simulink model "ipmsm_current_control_CV_FF"  (R2023a)
settings: Solver=FixedStepDiscrete  StartTime=0.0  StopTime=0.8  FixedStep=Ts  RelTol=1e-3  EnableMultiTasking=on
PreLoadFcn:
  | ee_ipmsm_velocity_control_data;
StopFcn:
  | ee_addSimlogTimeStamp(bdroot)
values from neighbouring files (symbols this model uses):
  ActCV = 1    [ipmsm_current_control_data.m]
  down1 = den(1)    [ipmsm_current_control_data.m]
  down2 = den(2)    [ipmsm_current_control_data.m]
  Ki_id = 0.6*Ld/(5*sigma*sigma)    (= 3750)    [ipmsm_current_control_data.m]
  Ki_iq = 0.6*Lq/(5*sigma*sigma)    (= 3750)    [ipmsm_current_control_data.m]
  Kp_id = 0.6*Ld/sigma    (= 1.5)    [ipmsm_current_control_data.m]
  Kp_iq = 0.6*Lq/sigma    (= 1.5)    [ipmsm_current_control_data.m]
  Ld = 0.2e-3    (= 0.0002)    [ipmsm_current_control_data.m]
  Lq = 0.2e-3    (= 0.0002)    [ipmsm_current_control_data.m]
  p = 4    [ipmsm_current_control_data.m]
  Pmax = 1.2*445.3845    (= 534.4614)    [ipmsm_current_control_data.m]
  psim = 0.0064    [ipmsm_current_control_data.m]
  Tmax = 1.2*0.8223    (= 0.98676)    [ipmsm_current_control_data.m]
  Ts = 1e-6    (= 1e-06)    [ipmsm_current_control_data.m]
  Tsi = 5e-5    (= 5e-05)    [ipmsm_current_control_data.m]
  up = num(2)    [ipmsm_current_control_data.m]
  Vnom = 24    [ipmsm_current_control_data.m]
undefined symbols (not defined in the file or in its folder): ee_sli_rtmsupport, gcbh, ID_MAP, IQ_MAP, RPM_VECT, TQ_VECT, VDC_VECT
libraries: nesl_utility x13, fl_lib x10, simulink x10, ee_lib x5, spsMeanLib x4, slpidlib x2, eeDiscretePi x2, eeTransforms x2, eeVelocityController x1, eePwmGeneratorTwoLevel x1, SignalEditorBlockLib x1
(part 1 of 2)
CloseFcn:
  | try,close(h1_ee_ipmsm_velocity_control),end
  | clear h1_ee_ipmsm_velocity_control
  | 
  | clear simlog_ee_ipmsm_velocity_control
  | clear logsout_ee_ipmsm_velocity_control
  | 
  | clear Pmax Tmax p psim Ld Lq L0 Rs Jm
  | clear Cdc Vnom V1 AH0
  | clear Ts fsw Tsi Tso Kp_id Ki_id Kp_iq Ki_iq
  | clear numd_id dend_id numd_iq dend_iq
  | clear Kp_omega Ki_omega numd_omega dend_omega
  | clear ID_MAP IQ_MAP RPM_VECT TQ_VECT VDC_VECT
Description:
  | IPMSM Velocity Control
settings Model: SimulationMode=accelerator  Creator=The MathWorks, Inc.  LastModifiedBy=zxzhu
settings SolverCC: AlgebraicLoopSolver=TrustRegion  AutoInsertRateTranBlk=on  MaxZcPerStep=1
settings DataIOCC: MaxDataPoints=210000  ReturnWorkspaceOutputs=off  SignalLoggingName=logsout_ee_ipmsm_velocity_control
settings OptimizationCC: ReuseModelBlockBuffer=off  LifeSpan=inf
settings DebuggingCC: UnderspecifiedInitializationDetection=Classic  MergeDetectMultiDrivingBlocksExec=none  UnconnectedInputMsg=warning  UnconnectedOutputMsg=warning  UnconnectedLineMsg=warning  SFUnexpectedBacktrackingDiag=warning  SFNoUnconditionalDefaultTransitionDiag=warning  SFExecutionAtInitializationDiag=none  ArithmeticOperatorsInVariantConditions=warning
settings ModelReferenceCC: EnableRefExpFcnMdlSchedulingChecks=on
settings SFSimCC: SimUseLocalCustomCode=off  CustomCodeUndefinedFunction=UseInterfaceOnly
settings RTWCC: RTWUseLocalCustomCode=off  DLArmComputeVersion=19.05
settings CodeAppCC: StateflowObjectComments=on
settings GRTTargetCC: TargetLangStandard=C89/C90 (ANSI)
settings ConfigComp: CovMetricSettings=dw  CovSaveCumulativeToWorkspaceVar=on  CovSaveSingleToWorkspaceVar=on  CovExternalEMLEnable=off
settings SimscapeCC: SimscapeNormalizeSystem=off  SimscapeLogType=all  SimscapeLogSimulationStatistics=on  SimscapeLogName=simlog_ee_ipmsm_velocity_control  SimscapeLogDataHistory=210000

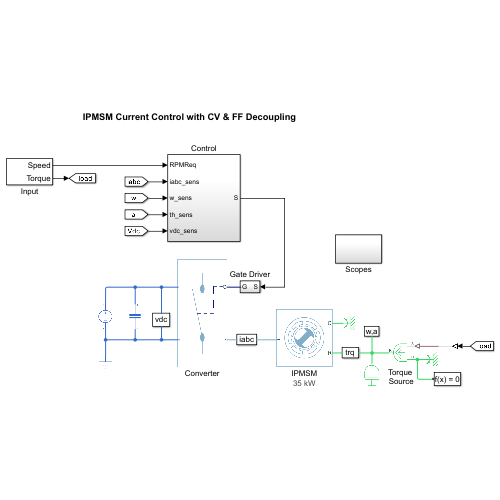
[thumbnail: Simulink's stored preview of the top-level diagram]
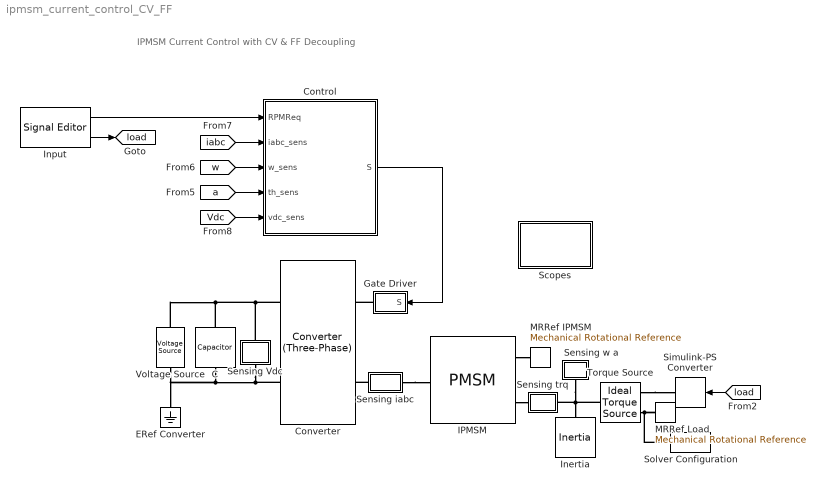
== system ipmsm_current_control_CV_FF ==
  note: IPMSM Current Control with CV & FF Decoupling
  C : fl_lib/Electrical/Electrical Elements/Capacitor  c=Cdc F  r=1e-6 Ohm  g=0 1/Ohm  i_specify=off  i_priority=None  i=0 A  i_nominal_specify=off  i_nominal_unit=A  i_nominal_value=1  v_specify=off  v_priority=None  v=0 V  v_nominal_specify=off  v_nominal_unit=V  v_nominal_value=1  vc_specify=on  vc_priority=None  vc=Vnom V  vc_nominal_specify=off  vc_nominal_unit=V  vc_nominal_value=1
  Control : Subsystem
  Converter : ee_lib/Semiconductors & Converters/Converters/Converter (Three-Phase)  port_option=ee.enum.threePhasePort.composite  device_type=3  K=0  Vf=0.8 V  Ron=0.001 Ohm  Rds=0.001 Ohm  Goff=1e-5 1/Ohm  Vgt=1 V  Vgt_off=-1 V  Ih=1 A  Vth=0.5 V  diode_param=2  diode_Vf=0.8 V  diode_Ron=0.001 Ohm  diode_Goff=1e-5 1/Ohm  diode_C=50 nF  diode_iRM=-235 A  diode_iF=300 A  diode_idot=-50 A/us  diode_trr_param=1  diode_trr_factor=3  diode_trr=15 us  diode_Qrr=1.5e+3 s*uA  snubber_type=0  Cs=1e-7 F  Rs=0.1 Ohm
  ERef Converter : fl_lib/Electrical/Electrical Elements/Electrical Reference
  Gate Driver : Subsystem
  IPMSM : ee_lib/Electromechanical/Permanent Magnet/PMSM  port_option=ee.enum.threePhasePort.composite  winding_type=ee.enum.statorconnection.wye  machine_param=ee.enum.pmsm.parameterization.constant  nPolePairs=p  pmflux_param=1  pm_flux_linkage=psim Wb  torque_constant=0.18 N*m/A  back_emf_constant=0.18 V/(rad/s)  stator_param=1  Ld=Ld H  Lq=Lq H  idVec=[-200, 0, 200] A  iqVec=[-200, 0, 200] A  LdMatrix=0.0002 * ones(3, 3) H  LqMatrix=0.0002 * ones(3, 3) H  PmMatrix=0.1 * ones(3, 3) Wb  ktMatrix=0.18 * ones(3, 3) N*m/A  keMatrix=0.18 * ones(3, 3) V/(rad/s)  L0=L0 H  Ls=0.0002 H  Lm=0.00002 H  Ms=0.00002 H  Rs=Rs Ohm  zero_sequence=ee.enum.park.zerosequence.exclude  axes_param=ee.enum.rotorangle.daxis  loss_param=ee.enum.ironloss.none  losses_oc=[0, 0, 0] W  losses_sc=[0, 0, 0] W  f_losses=60 Hz  Isc_losses=95 A  J=0 kg*m^2  lam=0 N*m/(rad/s)  i_d_specify=off  i_d_priority=None  i_d=0 A  i_d_nominal_specify=off  i_d_nominal_unit=A  i_d_nominal_value=1  i_q_specify=off  i_q_priority=None  i_q=0 A  i_q_nominal_specify=off  i_q_nominal_unit=A  i_q_nominal_value=1  torque_specify=off  torque_priority=None  torque=0 N*m  torque_nominal_specify=off  torque_nominal_unit=N*m  torque_nominal_value=1  angular_velocity_specify=on  angular_velocity_priority=None  angular_velocity=0 rpm  angular_velocity_nominal_specify=off  angular_velocity_nominal_unit=rpm  angular_velocity_nominal_value=1  angular_position_specify=on  angular_position_priority=High  angular_position=0 rad  angular_position_nominal_specify=off  angular_position_nominal_unit=deg  angular_position_nominal_value=1  alpha=3.93e-3 1/K  alpha_flux=-0.001 1/K  Tmeas=298.15 K  stator_thermal_mass=100 J/K  rotor_thermal_mass=200 J/K  Rm_percent_rotor=90  Rd_percent_rotor=30  temperatureA_specify=off  temperatureA_priority=High  temperatureA=25 degC  temperatureA_nominal_specify=off  temperatureA_nominal_unit=degC  temperatureA_nominal_value=1  temperatureB_specify=off  temperatureB_priority=High  temperatureB=25 degC  temperatureB_nominal_specify=off  temperatureB_nominal_unit=degC  temperatureB_nominal_value=1  temperatureC_specify=off  temperatureC_priority=High  temperatureC=25 degC  temperatureC_nominal_specify=off  temperatureC_nominal_unit=degC  temperatureC_nominal_value=1  temperatureR_specify=off  temperatureR_priority=High  temperatureR=25 degC  temperatureR_nominal_specify=off  temperatureR_nominal_unit=degC  temperatureR_nominal_value=1
      settings: AttributesFormatString=35 kW  InternalSimscapePortConfiguration="{\"Bottom\":[],\"Left\":[{\"id\":\"N\",\"label\":\"~\",\"type\":\"foundation.electrical.three_phase\"}],\"Right\":[{\"id\":\"R\",\"label\":\"R\",\"type\":\"foundation.mechanical.rotational.rotational\"},{\"id\":\"C\",\"label\":\"C\",\"type\":\"foundation.mechanical.rotational.rotational\"}],\"Top\":[]}"
  Inertia : fl_lib/Mechanical/Rotational Elements/Inertia  inertia=Jm kg*m^2  num_ports=foundation.enum.numPorts2.one  w_specify=on  w_priority=High  w=0 rpm  w_nominal_specify=off  w_nominal_unit=rad/s  w_nominal_value=1  t_specify=off  t_priority=High  t=0 N*m  t_nominal_specify=off  t_nominal_unit=N*m  t_nominal_value=1
  Input : SignalEditorBlockLib/Signal Editor  FileName=ipmsm_current_control_Input.mat  ActiveScenario=Test_2000rpm  ActiveSignal=Speed  IsBus=off  OutputBusObjectStr=Bus: BusObject  SampleTime=0  OutputAfterFinalValue=Extrapolation  Unit=inherit  PreserveSignalName=on  ApplySigPropsToAllScenarios=on
  MRRef IPMSM : fl_lib/Mechanical/Rotational Elements/Mechanical Rotational Reference
  MRRef Load : fl_lib/Mechanical/Rotational Elements/Mechanical Rotational Reference
  Scopes : Subsystem
  Sensing Vdc : Subsystem
      mask Display: disp('vdc')
  Sensing trq : Subsystem
      mask Display: disp('trq')
  Sensing w a : Subsystem
      mask Display: disp('w,a')
  Sensing iabc : Subsystem
      mask Display: disp('iabc')
  Simulink-PS Converter : nesl_utility/Simulink-PS Converter  PhysicalDomain=network_engine_domain  SubClassName=ps_input  LeftPortType=input  RightPortType=output  PseudoPeriodic=off  Frequencies=[]  NoiseDistribution=none  NoiseParameters=[]  Unit=N*m  AffineConversion=off  FilteringAndDerivatives=zero  SimscapeFilterOrder=1  InputFilterTimeConstant=0.001  UdotUserProvided=1
  Solver Configuration : nesl_utility/Solver Configuration  PhysicalDomain=network_engine_domain  SubClassName=solver  LeftPortType=input  RightPortType=generic  Tones=[]  Harmonics=[]  SimulateNoise=off  Profile=off  UseLocalSampling=off  EnableSwitchedLinearOptims=on  FrequencyDomain=off  UseCCode=off  RelTol=0.001  AbsTol=1e-06  MinStep=1e-09  ToWorkspace=off  RevertToSquareIcSolve=off  NumHomotopyIterations=100  PhasorMode=off  PhasorModeNumHarmonics=1  ConsistencySolver=NEWTON_FTOL  IndexReductionMethod=DerivativeReplacement  DoDC=off  ResidualTolerance=1e-9  ConsistencyTolSource=GLOBAL  ConsistencyAbsTol=0.001  ConsistencyRelTol=0.001  ConsistencyTolFactor=0.001  UseLocalSolver=on  LocalSolverChoice=NE_BACKWARD_EULER_ADVANCER  ResolveIndetEquations=on  FunctionEvalNumThread=1  LocalSolverSampleTime=Ts  DoFixedCost=on  MaxNonlinIter=5  MaxModeIter=2  ComputeImpulses=off  ImpulseIterations=2  LinearAlgebra=auto  LinearAlgebraNumThread=0  EquationFormulation=NE_TIME_EF  DelaysMemoryBudget=1024  AutomaticFiltering=on  FilteringTimeConstant=0.001  PartitionStorageMethod=AS_NEEDED  PartitionMemoryBudget=1024  PartitionMethod=FAST
  Torque Source : fl_lib/Mechanical/Mechanical Sources/Ideal Torque Source
  Voltage Source : ee_lib/Sources/Voltage Source  dc_voltage=Vnom V  ac_voltage=0 V  ac_shift=0 rad  ac_frequency=60 Hz  noise_mode=ee.enum.sources.noise.Disabled  PSD=0 V^2/Hz  sample_time=1e-3 s  repeatability=ee.enum.sources.repeatability.NotRepeatable  user_seed=0  auto_seed=3499211588  i_specify=off  i_priority=None  i=0 A  i_nominal_specify=off  i_nominal_unit=A  i_nominal_value=1  v_specify=off  v_priority=None  v=0 V  v_nominal_specify=off  v_nominal_unit=V  v_nominal_value=1
  tag scope: load=global
  wires:
  Control/1(S) -> Gate Driver/1(S)
  [load] -> Simulink-PS Converter/1
  [Vdc] -> Control/5(vdc_sens)
  [iabc] -> Control/2(iabc_sens)
  [w] -> Control/3(w_sens)
  [a] -> Control/4(th_sens)
  Input/2 -> [load]
  Input/1 -> Control/1(RPMReq)
  connections:
  Converter/RConn1 -- Sensing Vdc/LConn1 -- Voltage Source/LConn1 -- C/LConn1
  Torque Source/LConn1 -- Sensing trq/RConn1 -- Inertia/LConn1 -- Sensing w a/LConn1
  Gate Driver/RConn1 -- Converter/LConn1
  Torque Source/RConn1 -- Simulink-PS Converter/RConn1
  Torque Source/RConn2 -- Solver Configuration/RConn1 -- MRRef Load/LConn1
  Sensing iabc/LConn1 -- Converter/LConn2
  IPMSM/RConn2 -- MRRef IPMSM/LConn1
  IPMSM/RConn1 -- Sensing trq/LConn1
  Voltage Source/RConn1 -- ERef Converter/LConn1 -- Converter/RConn2 -- Sensing Vdc/RConn1 -- C/RConn1
  Sensing iabc/RConn1 -- IPMSM/LConn1

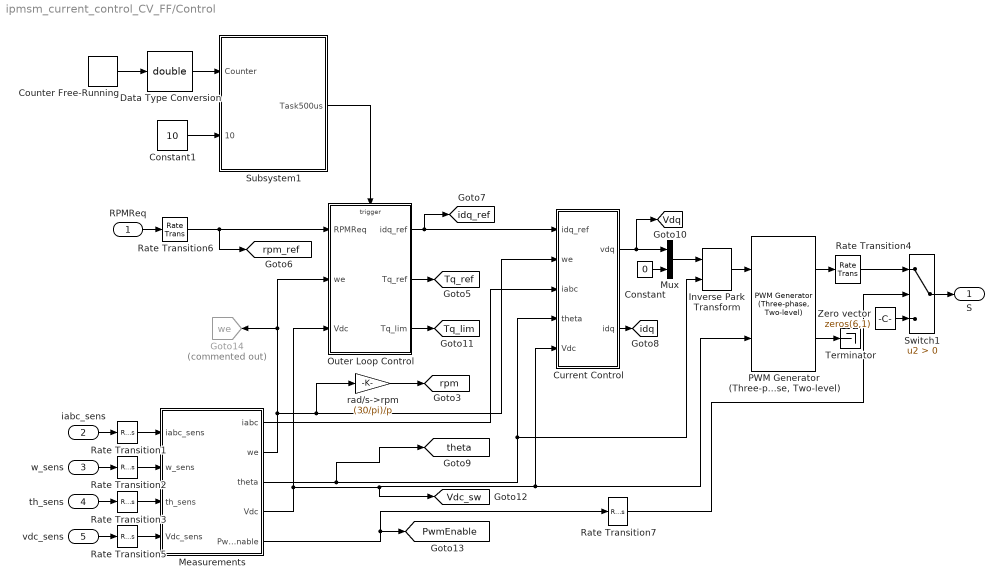
== system ipmsm_current_control_CV_FF/Control ==
  RPMReq : Inport
  iabc_sens : Inport  Port=2
  w_sens : Inport  Port=3
  th_sens : Inport  Port=4
  vdc_sens : Inport  Port=5
  Constant : Constant  Value=0  SampleTime=-1
  Constant1 : Constant  Value=10
  Counter Free-Running : simulink/Sources/Counter Free-Running  NumBits=32  tsamp=5e-5
  Current Control : Subsystem
  Data Type Conversion : DataTypeConversion  OutDataTypeStr=double  SaturateOnIntegerOverflow=off  RndMeth=Floor
  Goto14 : Goto  Commented=on  GotoTag=we  TagVisibility=global
  Inverse Park Transform : eeTransforms/Inverse Park Transform  AxisAlignment=D-axis  PowerInvariant=off
  Measurements : Subsystem
  Mux : Mux  Inputs=2
  Outer Loop Control : Subsystem
  "PWM Generator (Three-phase, Two-level)" : eePwmGeneratorTwoLevel/PWM Generator (Three-phase, Two-level)  PWMMode=Continuous PWM (CPWM)  CPWMMode=SVM: space vector modulation  DPWMMode=60 DPWM: 60 degree discontinuous PWM  fsw=fsw  Ts=Ts
      settings: SamplingMode=Asymmetric
  Rate Transition{1..7} (7 alike) : RateTransition
  Subsystem1 : Subsystem
  Switch1 : Switch  Criteria=u2 > Threshold  SaturateOnIntegerOverflow=off  InputSameDT=off
  Terminator : Terminator
  Zero vector : Constant  Value=zeros(6,1)
  rad/s->rpm : Gain  Gain=(30/pi)/p
  S : Outport  VectorParamsAs1DForOutWhenUnconnected=off
  tag scope: PwmEnable=global, Tq_lim=global, Tq_ref=global, Vdc_sw=global, Vdq=global, idq=global, idq_ref=global, rpm=global, rpm_ref=global, theta=global
  wires:
  Current Control/1(vdq) -> Mux/1, [Vdq]
  Measurements/1(iabc) -> Current Control/3(iabc)
  "PWM Generator (Three-phase, Two-level)"/1 -> Rate Transition4/1
  iabc_sens/1 -> Rate Transition1/1
  w_sens/1 -> Rate Transition2/1
  th_sens/1 -> Rate Transition3/1
  vdc_sens/1 -> Rate Transition5/1
  Outer Loop Control/1(idq_ref) -> [idq_ref], Current Control/1(idq_ref)
  RPMReq/1 -> Rate Transition6/1
  "PWM Generator (Three-phase, Two-level)"/2 -> Terminator/1
  Rate Transition1/1 -> Measurements/1(iabc_sens)
  Rate Transition2/1 -> Measurements/2(w_sens)
  Rate Transition3/1 -> Measurements/3(th_sens)
  Rate Transition5/1 -> Measurements/4(Vdc_sens)
  Rate Transition6/1 -> [rpm_ref], Outer Loop Control/1(RPMReq)
  Measurements/4(Vdc) -> Outer Loop Control/3(Vdc), [Vdc_sw], Current Control/5(Vdc), "PWM Generator (Three-phase, Two-level)"/2
  Outer Loop Control/2(Tq_ref) -> [Tq_ref]
  Measurements/2(we) -> Goto14/1, Outer Loop Control/2(we), Current Control/2(we), rad/s->rpm/1
  rad/s->rpm/1 -> [rpm]
  Current Control/2(idq) -> [idq]
  Outer Loop Control/3(Tq_lim) -> [Tq_lim]
  Switch1/1 -> S/1
  Rate Transition4/1 -> Switch1/1
  Measurements/5(PwmEnable) -> Rate Transition7/1, [PwmEnable]
  Zero vector/1 -> Switch1/3
  Rate Transition7/1 -> Switch1/2
  Mux/1 -> Inverse Park Transform/1
  Constant/1 -> Mux/2
  Constant1/1 -> Subsystem1/2(10)
  Counter Free-Running/1 -> Data Type Conversion/1
  Subsystem1/1(Task500us) -> Outer Loop Control/Trigger
  Data Type Conversion/1 -> Subsystem1/1(Counter)
  Inverse Park Transform/1 -> "PWM Generator (Three-phase, Two-level)"/1
  Measurements/3(theta) -> Current Control/4(theta), Inverse Park Transform/2, [theta]

== system ipmsm_current_control_CV_FF/Gate Driver ==
  S : Inport
  Demux : Demux  Outputs=6
  Simulink-PS Converter{1..6} (6 alike) : nesl_utility/Simulink-PS Converter  PhysicalDomain=network_engine_domain  SubClassName=ps_input  LeftPortType=input  RightPortType=output  PseudoPeriodic=off  Frequencies=[]  NoiseDistribution=none  NoiseParameters=[]  Unit=1  AffineConversion=off  FilteringAndDerivatives=zero  SimscapeFilterOrder=1  InputFilterTimeConstant=0.001  UdotUserProvided=1
  Six-Pulse Gate Multiplexer : ee_lib/Semiconductors & Converters/Converters/Six-Pulse Gate Multiplexer  port_option=ee.enum.controlport.ps
  G : PMIOPort  Side=Right
  wires:
  Demux/1 -> Simulink-PS Converter1/1
  S/1 -> Demux/1
  Demux/4 -> Simulink-PS Converter4/1
  Demux/2 -> Simulink-PS Converter2/1
  Demux/3 -> Simulink-PS Converter3/1
  Demux/5 -> Simulink-PS Converter5/1
  Demux/6 -> Simulink-PS Converter6/1
  connections:
  Six-Pulse Gate Multiplexer/RConn1 -- G/RConn1
  Simulink-PS Converter1/RConn1 -- Six-Pulse Gate Multiplexer/LConn1
  Simulink-PS Converter3/RConn1 -- Six-Pulse Gate Multiplexer/LConn3
  Simulink-PS Converter5/RConn1 -- Six-Pulse Gate Multiplexer/LConn5
  Simulink-PS Converter6/RConn1 -- Six-Pulse Gate Multiplexer/LConn6
  Simulink-PS Converter4/RConn1 -- Six-Pulse Gate Multiplexer/LConn4
  Simulink-PS Converter2/RConn1 -- Six-Pulse Gate Multiplexer/LConn2

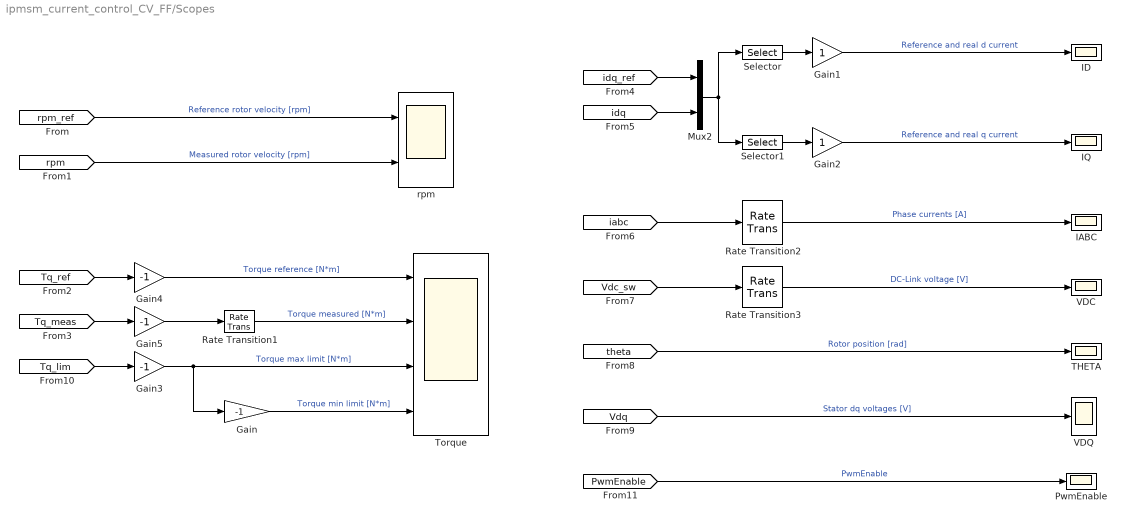
== system ipmsm_current_control_CV_FF/Scopes ==
  Gain{,3..5} (4 alike) : Gain  Gain=-1
  Gain1 : Gain
  Gain2 : Gain
  IABC : Scope
  ID : Scope
  IQ : Scope
  Mux2 : Mux  Inputs=2
  PwmEnable : Scope
  Rate Transition1 : RateTransition
  Rate Transition2 : RateTransition  OutPortSampleTime=1e-4
  Rate Transition3 : RateTransition  OutPortSampleTime=1e-4
  Selector : Selector  InputPortWidth=4  IndexOptions=Index vector (dialog)  Indices=[1 3]  OutputSizes=1
  Selector1 : Selector  InputPortWidth=4  IndexOptions=Index vector (dialog)  Indices=[2 4]  OutputSizes=1
  THETA : Scope
  Torque : Scope  NumInputPorts=4
  VDC : Scope
  VDQ : Scope
  rpm : Scope  NumInputPorts=2
  wires:
  [rpm] -> rpm/2  "Measured rotor velocity [rpm]"
  Mux2/1 -> Selector1/1, Selector/1
  Gain/1 -> Torque/4  "Torque min limit [N*m]"
  Rate Transition3/1 -> VDC/1  "DC-Link voltage [V]"
  [Vdc_sw] -> Rate Transition3/1
  [idq_ref] -> Mux2/1
  [PwmEnable] -> PwmEnable/1  "PwmEnable"
  [Tq_ref] -> Gain4/1
  Rate Transition2/1 -> IABC/1  "Phase currents [A]"
  [idq] -> Mux2/2
  [rpm_ref] -> rpm/1  "Reference rotor velocity [rpm]"
  [iabc] -> Rate Transition2/1
  [Tq_meas] -> Gain5/1
  [Vdq] -> VDQ/1  "Stator dq voltages [V]"
  [Tq_lim] -> Gain3/1
  [theta] -> THETA/1  "Rotor position [rad]"
  Rate Transition1/1 -> Torque/2  "Torque measured [N*m]"
  Selector/1 -> Gain1/1
  Selector1/1 -> Gain2/1
  Gain1/1 -> ID/1  "Reference and real d current"
  Gain2/1 -> IQ/1  "Reference and real q current"
  Gain3/1 -> Gain/1, Torque/3  "Torque max limit [N*m]"
  Gain4/1 -> Torque/1  "Torque reference [N*m]"
  Gain5/1 -> Rate Transition1/1

== system ipmsm_current_control_CV_FF/Sensing Vdc ==
  PS-Simulink Converter4 : nesl_utility/PS-Simulink Converter  PhysicalDomain=network_engine_domain  SubClassName=ps_output  LeftPortType=input  RightPortType=output  PseudoPeriodic=off  Frequencies=[]  VectorFormat=1-D array  Unit=V  AffineConversion=off
  Voltage Sensor : fl_lib/Electrical/Electrical Sensors/Voltage Sensor
  + : PMIOPort  Side=Left
  - : PMIOPort  Port=2  Side=Right
  tag scope: Vdc=global
  wires:
  PS-Simulink Converter4/1 -> [Vdc]
  connections:
  Voltage Sensor/LConn1 -- +/RConn1
  Voltage Sensor/RConn2 -- -/RConn1
  PS-Simulink Converter4/LConn1 -- Voltage Sensor/RConn1

== system ipmsm_current_control_CV_FF/Sensing trq ==
  PS-Simulink Converter3 : nesl_utility/PS-Simulink Converter  PhysicalDomain=network_engine_domain  SubClassName=ps_output  LeftPortType=input  RightPortType=output  PseudoPeriodic=off  Frequencies=[]  VectorFormat=1-D array  Unit=N*m  AffineConversion=off
  Torque Sensor : fl_lib/Mechanical/Mechanical Sensors/Ideal Torque Sensor
  R : PMIOPort  Side=Left
  C : PMIOPort  Port=2  Side=Right
  tag scope: Tq_meas=global
  wires:
  PS-Simulink Converter3/1 -> [Tq_meas]
  connections:
  Torque Sensor/RConn1 -- C/RConn1
  Torque Sensor/RConn2 -- PS-Simulink Converter3/LConn1
  Torque Sensor/LConn1 -- R/RConn1

== system ipmsm_current_control_CV_FF/Sensing w a ==
  MRRef : fl_lib/Mechanical/Rotational Elements/Mechanical Rotational Reference
  Motion Sensor : fl_lib/Mechanical/Mechanical Sensors/Ideal Rotational Motion Sensor  reference=foundation.enum.MeasurementReference.difference  acceleration_port=false  velocity_port=true  position_port=true  wrap_angle=simscape.enum.onoff.off  offset=0 deg
  PS-Simulink Converter1 : nesl_utility/PS-Simulink Converter  PhysicalDomain=network_engine_domain  SubClassName=ps_output  LeftPortType=input  RightPortType=output  PseudoPeriodic=off  Frequencies=[]  VectorFormat=1-D array  Unit=rad/s  AffineConversion=off
  PS-Simulink Converter2 : nesl_utility/PS-Simulink Converter  PhysicalDomain=network_engine_domain  SubClassName=ps_output  LeftPortType=input  RightPortType=output  PseudoPeriodic=off  Frequencies=[]  VectorFormat=1-D array  Unit=rad  AffineConversion=off
  R : PMIOPort  Side=Left
  tag scope: a=global, w=global
  wires:
  PS-Simulink Converter1/1 -> [w]
  PS-Simulink Converter2/1 -> [a]
  connections:
  R/RConn1 -- Motion Sensor/LConn1
  Motion Sensor/RConn2 -- PS-Simulink Converter1/LConn1
  MRRef/LConn1 -- Motion Sensor/RConn1
  Motion Sensor/RConn3 -- PS-Simulink Converter2/LConn1

== system ipmsm_current_control_CV_FF/Sensing iabc ==
  Current Sensor : ee_lib/Sensors & Transducers/Current Sensor (Three-Phase)
  PS-Simulink Converter : nesl_utility/PS-Simulink Converter  PhysicalDomain=network_engine_domain  SubClassName=ps_output  LeftPortType=input  RightPortType=output  PseudoPeriodic=off  Frequencies=[]  VectorFormat=1-D array  Unit=A  AffineConversion=off
  1 : PMIOPort  Side=Left
  2 : PMIOPort  Port=2  Side=Right
  tag scope: iabc=global
  wires:
  PS-Simulink Converter/1 -> [iabc]
  connections:
  1/RConn1 -- Current Sensor/LConn1
  2/RConn1 -- Current Sensor/RConn2
  Current Sensor/RConn1 -- PS-Simulink Converter/LConn1

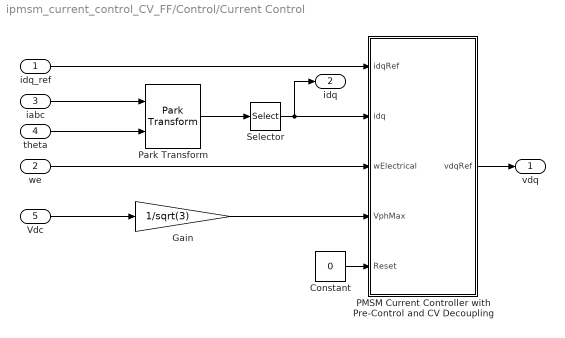
== system ipmsm_current_control_CV_FF/Control/Current Control ==
  idq_ref : Inport
  we : Inport  Port=2
  iabc : Inport  Port=3
  theta : Inport  Port=4
  Vdc : Inport  Port=5
  Constant : Constant  Value=0  SampleTime=-1
  Gain : Gain  Gain=1/sqrt(3)
  PMSM Current Controller with Pre-Control and CV Decoupling : Subsystem  AncestorBlock=eePmsmCurrentController/PMSM Current Controller with Pre-Control  LoadFcn=ee_sli_rtmsupport( 'loadfcn', gcbh );  mask(PMSM Current Controller with Pre-Control){Kp_id=Kp_id, Ki_id=Ki_id, Kaw_id=1, Kp_iq=Kp_iq, Ki_iq=Ki_iq, Kaw_iq=1, Ts=-1, Tsd=Tsi, AxisPrio=Q-axis, ActZC=on, ActFF=on, idVect=[-200, 0, 200], iqVect=[-200, 0, 200], LdMatrix=Ld * ones(3, 3), LqMatrix=Lq * ones(3, 3), psimMatrix=psim * ones(3, 3)}
      mask prompts: Kp_id "physmod:ee:library:comments:control:eePmsmCurrentController:DaxisCurrentProportionalGain_MP"; Ki_id "physmod:ee:library:comments:control:eePmsmCurrentController:DaxisCurrentIntegralGain_MP"; Kaw_id "physmod:ee:library:comments:control:eePmsmCurrentController:DaxisCurrentAntiwindupGain_MP"; Kp_iq "physmod:ee:library:comments:control:eePmsmCurrentController:QaxisCurrentProportionalGain_MP"; Ki_iq "physmod:ee:library:comments:control:eePmsmCurrentController:QaxisCurrentIntegralGain_MP"; Kaw_iq "physmod:ee:library:comments:control:eePmsmCurrentController:QaxisCurrentAntiwindupGain_MP"; Ts "physmod:ee:library:comments:control:eePmsmCurrentController:SampleTime1ForInherited_MP"; Tsd "physmod:ee:library:comments:control:eePmsmCurrentController:DiscretizationSampleTime_MP"; AxisPrio "physmod:ee:library:comments:control:eePmsmCurrentController:AxisPrioritization_MP"; ActZC "physmod:ee:library:comments:control:eePmsmCurrentController:EnableZeroCancellation_MP"; ActFF "physmod:ee:library:comments:control:eePmsmCurrentController:EnablePrecontrolVoltage_MP"; idVect "physmod:ee:library:comments:control:eePmsmCurrentController:DaxisCurrentVectorIdA_MP"; iqVect "physmod:ee:library:comments:control:eePmsmCurrentController:QaxisCurrentVectorIqA_MP"; LdMatrix "physmod:ee:library:comments:control:eePmsmCurrentController:LdMatrixLdidiqH_MP"; LqMatrix "physmod:ee:library:comments:control:eePmsmCurrentController:LqMatrixLqidiqH_MP"; psimMatrix "physmod:ee:library:comments:control:eePmsmCurrentController:PermanentMagnetFluxLinkageMatrixPMidiqWb_MP"
      mask help: physmod:ee:library:comments:control:eePmsmCurrentController:PMSMCurrentControllerWithPreControl_MD
      mask init:
      | [Tsd, numZC_id, denZC_id, numZC_iq, denZC_iq] = ee.mask.initializePmsmCurrentController(ActZC,Ts,Tsd,Kp_id,Ki_id,Kp_iq,Ki_iq);
      | 
      | if length(idVect) < 2            
      | 	error(message('physmod:simscape:compiler:patterns:checks:LengthGreaterThanOrEqual',getString(message('physmod:ee:library:comments:control:eePmsmCurrentController:DaxisCurrentVectorIdA_MP')), '2'));            
      | end
      | if ~all(diff(idVect) > 0)            
      | 	error(message('physmod:simscape:compiler:patterns:checks:StrictlyAscendingVec',getString(message('physmod:ee:library:comments:control:eePmsmCurrentController:DaxisCurrentVectorIdA_MP'))));            
      | end
      | if length(iqVect) < 2            
      | 	error(message('physmod:simscape:compiler:patterns:checks:LengthGreaterThanOrEqual',getString(message('physmod:ee:library:comments:control:eePmsmCurrentController:QaxisCurrentVectorIqA_MP')), '2'));            
      | end
      | if ~all(diff(iqVect) > 0)            
      | 	error(message('physmod:simscape:compiler:patterns:checks:StrictlyAscendingVec',getString(message('physmod:ee:library:comments:control:eePmsmCurrentController:QaxisCurrentVectorIqA_MP'))));            
      | end
      | if ~all(size(LdMatrix) == [length(idVect), length(iqVect)])            
      | 	error(message('physmod:simscape:compiler:patterns:checks:Size2DEqual',getString(message('physmod:ee:library:comments:control:eePmsmCurrentController:LdMatrixLdidiqH_MP')), getString(message('physmod:ee:library:comments:control:eePmsmCurrentController:DaxisCurrentVectorIdA_MP')), getString(message('physmod:ee:library:comments:control:eePmsmCurrentController:QaxisCurrentVectorIqA_MP'))));            
      | end
      | if ~all(size(LqMatrix) == [length(idVect), length(iqVect)])            
      | 	error(message('physmod:simscape:compiler:patterns:checks:Size2DEqual',getString(message('physmod:ee:library:comments:control:eePmsmCurrentController:LqMatrixLqidiqH_MP')), getString(message('physmod:ee:library:comments:control:eePmsmCurrentController:DaxisCurrentVectorIdA_MP')), getString(message('physmod:ee:library:comments:control:eePmsmCurrentController:QaxisCurrentVectorIqA_MP'))));            
      | end
      | if ~all(size(psimMatrix) == [length(idVect), length(iqVect)])            
      | 	error(message('physmod:simscape:compiler:patterns:checks:Size2DEqual',getString(message('physmod:ee:library:comments:control:eePmsmCurrentController:PermanentMagnetFluxLinkageMatrixPMidiqWb_MP')), getString(message('physmod:ee:library:comments:control:eePmsmCurrentController:DaxisCurrentVectorIdA_MP')), getString(message('physmod:ee:library:comments:control:eePmsmCurrentController:QaxisCurrentVectorIqA_MP'))));            
      | end
      settings: CopyFcn=ee_sli_rtmsupport( 'copyfcn', gcbh );  DeleteFcn=ee_sli_rtmsupport( 'deletefcn', gcbh );  ModelCloseFcn=ee_sli_rtmsupport( 'modelclosefcn', gcbh );  PostSaveFcn=ee_sli_rtmsupport( 'postsavefcn', gcbh );  PreCopyFcn=ee_sli_rtmsupport( 'precopyfcn', gcbh );  OpenFcn=ee_sli_rtmsupport( 'openfcn', gcbh );  CloseFcn=ee_sli_rtmsupport( 'closefcn', gcbh );  PreDeleteFcn=ee_sli_rtmsupport( 'predeletefcn', gcbh );
      mask Help: web(nesl_help(gcbh))
      mask Callback Ts: ee.mask.callbackZeroCancellation(gcb);
      mask TypeOptions AxisPrio: d-q Voltage Limiter/AxisPrio
      mask Callback ActZC: ee.mask.callbackZeroCancellation(gcb);
      mask Callback ActFF: ee.mask.callbackPmsmPreControl(gcb);
      mask DialogControl Container3 Prompt: physmod:ee:library:comments:control:eePmsmCurrentController:tab_ControlParameters
      mask DialogControl Kp_id Prompt: D-axis current proportional gain
      mask DialogControl Ki_id Prompt: D-axis current integral gain
      mask DialogControl Kaw_id Prompt: D-axis current anti-windup gain
      mask DialogControl Kp_iq Prompt: Q-axis current proportional gain
      mask DialogControl Ki_iq Prompt: Q-axis current integral gain
      mask DialogControl Kaw_iq Prompt: Q-axis current anti-windup gain
      mask DialogControl Ts Prompt: Sample time (-1 for inherited)
      mask DialogControl Tsd Prompt: Discretization sample time
      mask DialogControl AxisPrio Prompt: Axis prioritization
      mask DialogControl ActZC Prompt: Enable zero cancellation
      mask DialogControl ActFF Prompt: Enable pre-control voltage
      mask DialogControl Container4 Prompt: physmod:ee:library:comments:control:eePmsmCurrentController:tab_PreControlParameters
      mask DialogControl idVect Prompt: D-axis current vector, id (A)
      mask DialogControl iqVect Prompt: Q-axis current vector, iq (A)
      mask DialogControl LdMatrix Prompt: Ld matrix, Ld(id,iq), (H)
      mask DialogControl LqMatrix Prompt: Lq matrix, Lq(id,iq), (H)
      mask DialogControl psimMatrix Prompt: Permanent magnet flux linkage matrix, PM(id,iq), (Wb)
  Park Transform : eeTransforms/Park Transform  AxisAlignment=D-axis  PowerInvariant=off
  Selector : Selector  InputPortWidth=3  IndexOptions=Index vector (dialog)  Indices=[1 2]  OutputSizes=1
  vdq : Outport  VectorParamsAs1DForOutWhenUnconnected=off
  idq : Outport  Port=2  VectorParamsAs1DForOutWhenUnconnected=off
  wires:
  Vdc/1 -> Gain/1
  iabc/1 -> Park Transform/1
  we/1 -> PMSM Current Controller with Pre-Control and CV Decoupling/3(wElectrical)
  theta/1 -> Park Transform/2
  PMSM Current Controller with Pre-Control and CV Decoupling/1(vdqRef) -> vdq/1
  idq_ref/1 -> PMSM Current Controller with Pre-Control and CV Decoupling/1(idqRef)
  Constant/1 -> PMSM Current Controller with Pre-Control and CV Decoupling/5(Reset)
  Selector/1 -> idq/1, PMSM Current Controller with Pre-Control and CV Decoupling/2(idq)
  Gain/1 -> PMSM Current Controller with Pre-Control and CV Decoupling/4(VphMax)
  Park Transform/1 -> Selector/1

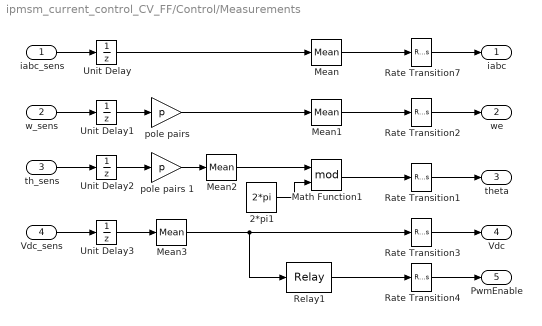
== system ipmsm_current_control_CV_FF/Control/Measurements ==
  iabc_sens : Inport
  w_sens : Inport  Port=2
  th_sens : Inport  Port=3
  Vdc_sens : Inport  Port=4
  2*pi1 : Constant  Value=2*pi  SampleTime=-1
  Math Function1 : Math  Operator=mod  SignedPower=on
  Mean{,1..3} (4 alike) : spsMeanLib/Mean  Freq=1/Tsi  Vinit=0  Ts=Ts
  Rate Transition{1..4,7} (5 alike) : RateTransition
  Relay1 : Relay  OnSwitchValue=.9*Vnom  OffSwitchValue=.8*Vnom
  Unit Delay{,1..3} (4 alike) : UnitDelay  SampleTime=2*Ts  HasFrameUpgradeWarning=on
  pole pairs : Gain  Gain=p
  pole pairs 1 : Gain  Gain=p
  iabc : Outport  VectorParamsAs1DForOutWhenUnconnected=off
  we : Outport  Port=2  VectorParamsAs1DForOutWhenUnconnected=off
  theta : Outport  Port=3  VectorParamsAs1DForOutWhenUnconnected=off
  Vdc : Outport  Port=4  VectorParamsAs1DForOutWhenUnconnected=off
  PwmEnable : Outport  Port=5  VectorParamsAs1DForOutWhenUnconnected=off
  wires:
  Mean2/1 -> Math Function1/1
  Mean1/1 -> Rate Transition2/1
  Mean/1 -> Rate Transition7/1
  Unit Delay1/1 -> pole pairs/1
  Unit Delay3/1 -> Mean3/1
  Unit Delay2/1 -> pole pairs 1/1
  iabc_sens/1 -> Unit Delay/1
  w_sens/1 -> Unit Delay1/1
  Unit Delay/1 -> Mean/1
  Vdc_sens/1 -> Unit Delay3/1
  pole pairs 1/1 -> Mean2/1
  th_sens/1 -> Unit Delay2/1
  pole pairs/1 -> Mean1/1
  Relay1/1 -> Rate Transition4/1
  Mean3/1 -> Rate Transition3/1, Relay1/1
  Math Function1/1 -> Rate Transition1/1
  2*pi1/1 -> Math Function1/2
  Rate Transition7/1 -> iabc/1
  Rate Transition1/1 -> theta/1
  Rate Transition2/1 -> we/1
  Rate Transition3/1 -> Vdc/1
  Rate Transition4/1 -> PwmEnable/1

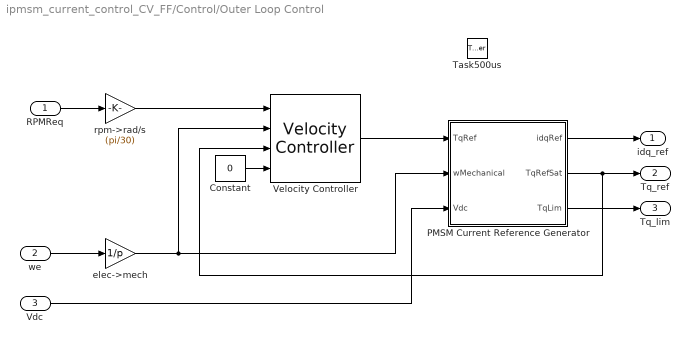
== system ipmsm_current_control_CV_FF/Control/Outer Loop Control ==
  RPMReq : Inport
  we : Inport  Port=2
  Vdc : Inport  Port=3
  Task500us : TriggerPort  VariantControl=Variant  PortDimensions=1
  Constant : Constant  Value=0  SampleTime=-1
  PMSM Current Reference Generator : Subsystem  AncestorBlock=eePmsmCurrentReferenceGen/PMSM Current Reference Generator  LoadFcn=ee_sli_rtmsupport( 'loadfcn', gcbh );  mask(PMSM Current Reference Generator){Vnom=Vnom, Pmax=Pmax, Tmax=Tmax, Ts=-1, RefType=Lookup-table based, rpmVec=RPM_VECT, TqVec=TQ_VECT, VdcVec=VDC_VECT, PWMMode=SVM: space vector modulation, ModFactor=1, idMatrix=ID_MAP, iqMatrix=IQ_MAP, p=8, psim=0.04, Ld=0.00024, Lq=0.00029, Rs=0.01, RefExpEnable=0}
      mask prompts: Vnom "physmod:ee:library:comments:control:eePmsmCurrentReferenceGen:NominalDclinkVoltageV_MP"; Pmax "physmod:ee:library:comments:control:eePmsmCurrentReferenceGen:MaximumPowerW_MP"; Tmax "physmod:ee:library:comments:control:eePmsmCurrentReferenceGen:MaximumTorqueNm_MP"; Ts "physmod:ee:library:comments:control:eePmsmCurrentReferenceGen:SampleTime1ForInherited_MP"; RefType "physmod:ee:library:comments:control:eePmsmCurrentReferenceGen:CurrentReferences_MP"; rpmVec "physmod:ee:library:comments:control:eePmsmCurrentReferenceGen:MechanicalSpeedVectorWMechanicalrpm_MP"; TqVec "physmod:ee:library:comments:control:eePmsmCurrentReferenceGen:TorqueReferenceVectorTqRefNm_MP"; VdcVec "physmod:ee:library:comments:control:eePmsmCurrentReferenceGen:DClinkVoltageVectorVdcV_MP"; PWMMode "physmod:ee:library:comments:control:eePmsmCurrentReferenceGen:PWMMethod_MP"; ModFactor "physmod:ee:library:comments:control:eePmsmCurrentReferenceGen:ModulationFactor_MP"; idMatrix "physmod:ee:library:comments:control:eePmsmCurrentReferenceGen:DaxisCurrentReferenceMatrixIdwMechanicalTqRefVdcA_MP"; iqMatrix "physmod:ee:library:comments:control:eePmsmCurrentReferenceGen:QaxisCurrentReferenceMatrixIqwMechanicalTqRefVdcA_MP"; p "physmod:ee:library:comments:control:eePmsmCurrentReferenceGen:NumberOfRotorPolePairs_MP"; psim "physmod:ee:library:comments:control:eePmsmCurrentReferenceGen:PermanentMagnetFluxLinkageWb_MP"; Ld "physmod:ee:library:comments:control:eePmsmCurrentReferenceGen:DaxisInductanceH_MP"; Lq "physmod:ee:library:comments:control:eePmsmCurrentReferenceGen:QaxisInductanceH_MP"; Rs "physmod:ee:library:comments:control:eePmsmCurrentReferenceGen:StatorResistanceOhm_MP"; RefExpEnable "physmod:ee:library:comments:control:eePmsmCurrentReferenceGen:ExportCurrentReferences_MP"
      mask help: physmod:ee:library:comments:control:eePmsmCurrentReferenceGen:PMSMCurrentReferenceGenerator_MD
      mask init:
      | if Vnom <= 0            
      |     error(message('physmod:simscape:compiler:patterns:checks:GreaterThanZero',getString(message('physmod:ee:library:comments:control:eePmsmCurrentReferenceGen:NominalDclinkVoltageV_MP'))));            
      | end
      | if Pmax <= 0            
      |     error(message('physmod:simscape:compiler:patterns:checks:GreaterThanZero',getString(message('physmod:ee:library:comments:control:eePmsmCurrentReferenceGen:MaximumPowerW_MP'))));            
      | end
      | if Tmax <= 0            
      |     error(message('physmod:simscape:compiler:patterns:checks:GreaterThanZero',getString(message('physmod:ee:library:comments:control:eePmsmCurrentReferenceGen:MaximumTorqueNm_MP'))));            
      | end
      | switch RefType
      |     case 'Zero d-axis control'
      |         EnableZDAC = 1;
      |         rpmVec = [0, 3000];
      |         TqVec  = [-100, 0, 100];
      |         VdcVec = [300, 350];
      |         idMatrix = zeros(2,3,2);
      |         iqMatrix = zeros(2,3,2);
      |     case 'Lookup-table based'
      |         EnableZDAC = 0;
      |         if length(rpmVec) < 2            
      |             error(message('physmod:simscape:compiler:patterns:checks:LengthGreaterThanOrEqual',getString(message('physmod:ee:library:comments:control:eePmsmCurrentReferenceGen:MechanicalSpeedVectorWMechanicalrpm_MP')), '2'));            
      |         end
      |         if ~all(diff(rpmVec) > 0)            
      |             error(message('physmod:simscape:compiler:patterns:checks:StrictlyAscendingVec',getString(message('physmod:ee:library:comments:control:eePmsmCurrentReferenceGen:MechanicalSpeedVectorWMechanicalrpm_MP'))));            
      |         end
      |         if length(TqVec) < 2            
      |             error(message('physmod:simscape:compiler:patterns:checks:LengthGreaterThanOrEqual',getString(message('physmod:ee:library:comments:control:eePmsmCurrentReferenceGen:TorqueReferenceVectorTqRefNm_MP')), '2'));            
      |         end
      |         if ~all(diff(TqVec) > 0)            
      |             error(message('physmod:simscape:compiler:patterns:checks:StrictlyAscendingVec',getString(message('physmod:ee:library:comments:control:eePmsmCurrentReferenceGen:TorqueReferenceVectorTqRefNm_MP'))));            
      |         end
      |         if length(VdcVec) < 2            
      |             error(message('physmod:simscape:compiler:patterns:checks:LengthGreaterThanOrEqual',getString(message('physmod:ee:library:comments:control:eePmsmCurrentReferenceGen:DClinkVoltageVectorVdcV_MP')), '2'));            
      |         end
      |         if ~all(diff(VdcVec) > 0)            
      |             error(message('physmod:simscape:compiler:patterns:checks:StrictlyAscendingVec',getString(message('physmod:ee:library:comments:control:eePmsmCurrentReferenceGen:DClinkVoltageVectorVdcV_MP'))));            
      |         end
      |         if ~all(size(idMatrix) == [length(rpmVec), length(TqVec), length(VdcVec)])            
      |             error(message('physmod:simscape:compiler:patterns:checks:Size3DEqual',getString(message('physmod:ee:library:comments:control:eePmsmCurrentReferenceGen:DaxisCurrentReferenceMatrixIdwMechanicalTqRefVdcA_MP')), getString(message('physmod:ee:library:comments:control:eePmsmCurrentReferenceGen:MechanicalSpeedVectorWMechanicalrpm_MP')), getString(message('physmod:ee:library:comments:control:eePmsmCurrentReferenceGen:TorqueReferenceVectorTqRefNm_MP')), getString(message('physmod:ee:library:comments:control:eePmsmCurrentReferenceGen:DClinkVoltageVectorVdcV_MP'))));            
      |         end
      |         if ~all(size(iqMatrix) == [length(rpmVec), length(TqVec), length(VdcVec)])            
      |             error(message('physmod:simscape:compiler:patterns:checks:Size3DEqual',getString(message('physmod:ee:library:comments:control:eePmsmCurrentReferenceGen:QaxisCurrentReferenceMatrixIqwMechanicalTqRefVdcA_MP')), getString(message('physmod:ee:library:comments:control:eePmsmCurrentReferenceGen:MechanicalSpeedVectorWMechanicalrpm_MP')), getString(message('physmod:ee:library:comments:control:eePmsmCurrentReferenceGen:TorqueReferenceVectorTqRefNm_MP')), getString(message('physmod:ee:library:comments:control:eePmsmCurrentReferenceGen:DClinkVoltageVectorVdcV_MP'))));            
      |         end
      |     case 'Automatically generated lookup-table'
      |         EnableZDAC = 0;
      |         if Rs <= 0            
      |             error(message('physmod:simscape:compiler:patterns:checks:GreaterThanZero',getString(message('physmod:ee:library:comments:control:eePmsmCurrentReferenceGen:StatorResistanceOhm_MP'))));            
      |         end
      |         if Ld <= 0            
      |             error(message('physmod:simscape:compiler:patterns:checks:GreaterThanZero',getString(message('physmod:ee:library:comments:control:eePmsmCurrentReferenceGen:DaxisInductanceH_MP'))));            
      |         end
      |         if Lq <= 0            
      |             error(message('physmod:simscape:compiler:patterns:checks:GreaterThanZero',getString(message('physmod:ee:library:comments:control:eePmsmCurrentReferenceGen:QaxisInductanceH_MP'))));            
      |         end
      |         
      |         if ModFactor <= 0            
      |             error(message('physmod:simscape:compiler:patterns:checks:GreaterThanZero',getString(message('physmod:ee:library:comments:control:eePmsmCurrentReferenceGen:ModulationFactor_MP'))));            
      |         end
      |         
      |         if ModFactor > 1            
      |             error(message('physmod:simscape:compiler:patterns:checks:LessThanOrEqual',getString(message('physmod:ee:library:comments:control:eePmsmCurrentReferenceGen:ModulationFactor_MP')),'1'));            
      |         end
      |         
      |         % Check if machine parameters were changed
      |         if exist('pmsm_data', 'var')
      |             dataUpdate = (pmsm_data.Ld   ~= Ld)   ||...
      |                          (pmsm_data.Lq   ~= Lq)   ||...
      |                          (pmsm_data.psim ~= psim) ||...
      |                          (pmsm_data.p    ~= p)    ||...
      |                          (pmsm_data.Rs   ~= Rs)   ||...
      |                          (pmsm_data.Pmax ~= Pmax) ||...
      |                          (pmsm_data.Tmax ~= Tmax) ||...
      |                          (pmsm_data.PWMMode ~= PWMMode) ||...
      |                          (pmsm_data.ModFactor ~= ModFactor);
      |         end
      |         % Check if grid points were changed
      |         if exist('grid_points', 'var')
      |             VecUpdate = max(abs(grid_points.RPM_VECT - rpmVec))~=0 ||...
      |                         max(abs(grid_points.TQ_VECT  - TqVec)) ~=0 ||...
      |                         max(abs(grid_points.VDC_VECT - VdcVec))~=0;
      |         end
      |         % Compute current references only IF current references do not exist OR 
      |         % machine parameters were changed OR grid points were changed
      |         if ~exist('pmsm_ref', 'var') || dataUpdate || VecUpdate
      |             grid_points.RPM_VECT = rpmVec;
      |             grid_points.TQ_VECT  = TqVec;
      |             grid_points.VDC_VECT = VdcVec;
      |             pmsm_data.Ld    = Ld; 
      |             pmsm_data.Lq    = Lq; 
      |             pmsm_data.psim  = psim;   
      |             pmsm_data.p     = p;         
      |             pmsm_data.Rs    = Rs;   
      |             pmsm_data.Pmax  = Pmax;      
      |             pmsm_data.Tbase = Tmax;    
      |             pmsm_data.PWMMode   = PWMMode;      
      |             pmsm_data.ModFactor = ModFactor;
      |             pmsm_ref = ee.control.pmsm.getCurrentReferencesPmsm ( pmsm_data, grid_points );
      |             idMatrix = pmsm_ref.idMatrix;
      |             iqMatrix = pmsm_ref.iqMatrix;
      |         end
      |         % Export current references to base workspace
      |         if RefExpEnable==1
      |             assignin('base', 'pmsm_ref', pmsm_ref)
      |             set_param(gcb,'RefExpEnable','0');
      |         end
      | end
      settings: CopyFcn=ee_sli_rtmsupport( 'copyfcn', gcbh );  DeleteFcn=ee_sli_rtmsupport( 'deletefcn', gcbh );  ModelCloseFcn=ee_sli_rtmsupport( 'modelclosefcn', gcbh );  PostSaveFcn=ee_sli_rtmsupport( 'postsavefcn', gcbh );  PreCopyFcn=ee_sli_rtmsupport( 'precopyfcn', gcbh );  OpenFcn=ee_sli_rtmsupport( 'openfcn', gcbh );  CloseFcn=ee_sli_rtmsupport( 'closefcn', gcbh );  PreDeleteFcn=ee_sli_rtmsupport( 'predeletefcn', gcbh );
      mask Help: web(nesl_help(gcbh))
      mask TypeOptions RefType: physmod:ee:library:comments:control:eePmsmCurrentReferenceGen:ZeroD0x2DAxisControl_PV | physmod:ee:library:comments:control:eePmsmCurrentReferenceGen:Lookup0x2DTableBased_PV | physmod:ee:library:comments:control:eePmsmCurrentReferenceGen:AutomaticallyGeneratedLookup0x2DTable_PV
      mask Callback RefType:
      | % Callback function to set the parameters visibility
      | ee.mask.callbackPopupRefGenPmsm(gcb);
      mask TypeOptions PWMMode: physmod:ee:library:comments:control:eePmsmCurrentReferenceGen:SPWMSinusoidalPWM_PV | physmod:ee:library:comments:control:eePmsmCurrentReferenceGen:SVMSpaceVectorModulation_PV
      mask DialogControl Container2 Prompt: physmod:ee:library:comments:control:eePmsmCurrentReferenceGen:tab_GeneralParameters
      mask DialogControl Vnom Prompt: Nominal dc-link voltage (V)
      mask DialogControl Pmax Prompt: Maximum power (W)
      mask DialogControl Tmax Prompt: Maximum torque (N*m)
      mask DialogControl Ts Prompt: Sample time (-1 for inherited)
      mask DialogControl Container3 Prompt: physmod:ee:library:comments:control:eePmsmCurrentReferenceGen:tab_ReferenceGenStrategy
      mask DialogControl RefType Prompt: Current references
      mask DialogControl rpmVec Prompt: Mechanical speed vector, wMechanical (rpm)
      mask DialogControl TqVec Prompt: Torque reference vector, TqRef (N*m)
      mask DialogControl VdcVec Prompt: DC-link voltage vector, Vdc (V)
      mask DialogControl PWMMode Prompt: PWM method
      mask DialogControl ModFactor Prompt: Modulation factor
      mask DialogControl idMatrix Prompt: D-axis current reference matrix, id(wMechanical,TqRef,Vdc), (A)
      mask DialogControl iqMatrix Prompt: Q-axis current reference matrix, iq(wMechanical,TqRef,Vdc), (A)
      mask DialogControl p Prompt: Number of rotor pole pairs
      mask DialogControl psim Prompt: Permanent magnet flux linkage (Wb)
      mask DialogControl Ld Prompt: D-axis inductance (H)
      mask DialogControl Lq Prompt: Q-axis inductance (H)
      mask DialogControl Rs Prompt: Stator resistance (Ohm)
      mask DialogControl RefExp Prompt: physmod:ee:library:comments:control:eePmsmCurrentReferenceGen:ExportCurrentReferencesToWorkspace_B
      mask DialogControl RefExp Callback:
      | % Enable export of current references
      | set_param(gcb,'RefExpEnable','1');
      mask DialogControl RefExpEnable Prompt: Export current references
  Velocity Controller : eeVelocityController/Velocity Controller  CtrlType=P-PI control  Kp_w=Kp_omega  Ki_w=Ki_omega  Kv_w=Kp_omega  Kaw_w=100  Ts=-1  Tsd=Tso  ActZC=on
  elec->mech : Gain  Gain=1/p
  rpm->rad/s : Gain  Gain=(pi/30)
  idq_ref : Outport  VectorParamsAs1DForOutWhenUnconnected=off
  Tq_ref : Outport  Port=2  VectorParamsAs1DForOutWhenUnconnected=off
  Tq_lim : Outport  Port=3  VectorParamsAs1DForOutWhenUnconnected=off
  wires:
  rpm->rad/s/1 -> Velocity Controller/1
  Velocity Controller/1 -> PMSM Current Reference Generator/1(TqRef)
  RPMReq/1 -> rpm->rad/s/1
  we/1 -> elec->mech/1
  Vdc/1 -> PMSM Current Reference Generator/3(Vdc)
  PMSM Current Reference Generator/1(idqRef) -> idq_ref/1
  PMSM Current Reference Generator/2(TqRefSat) -> Tq_ref/1, Velocity Controller/3
  PMSM Current Reference Generator/3(TqLim) -> Tq_lim/1
  elec->mech/1 -> PMSM Current Reference Generator/2(wMechanical), Velocity Controller/2
  Constant/1 -> Velocity Controller/4

== system ipmsm_current_control_CV_FF/Control/Subsystem1 ==
  Counter : Inport
  10 : Inport  Port=2
  Constant4 : Constant  Value=0
  Equal1 : RelationalOperator  Operator===  OutDataTypeStr=boolean  RndMeth=Simplest  InputSameDT=off
  Mod1 : Math  Operator=mod
  Task500us : Outport
  wires:
  Counter/1 -> Mod1/1
  10/1 -> Mod1/2
  Equal1/1 -> Task500us/1
  Mod1/1 -> Equal1/1
  Constant4/1 -> Equal1/2

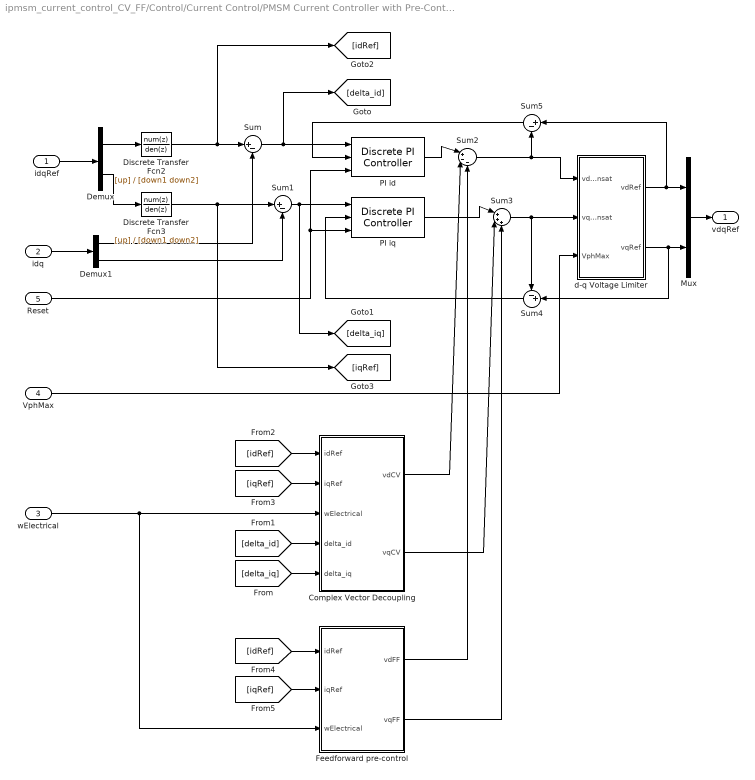
== system ipmsm_current_control_CV_FF/Control/Current Control/PMSM Current Controller with Pre-Control and CV Decoupling ==
  idqRef : Inport  SampleTime=Ts
  idq : Inport  Port=2  SampleTime=Ts
  wElectrical : Inport  Port=3  SampleTime=Ts
  VphMax : Inport  Port=4  SampleTime=Ts
  Reset : Inport  Port=5  SampleTime=Ts
  Complex Vector Decoupling : Subsystem
  Demux : Demux  Outputs=2
  Demux1 : Demux  Outputs=2
  Discrete Transfer Fcn2 : DiscreteTransferFcn  Numerator=[up]  Denominator=[down1 down2]
  Discrete Transfer Fcn3 : DiscreteTransferFcn  Numerator=[up]  Denominator=[down1 down2]
  Feedforward pre-control : Subsystem
  Mux : Mux  Inputs=2
  PI id : eeDiscretePi/Discrete PI Controller  Kp=Kp_id  Ki=Ki_id  Kaw=Kaw_id  x0=0  Ts=Ts
  PI iq : eeDiscretePi/Discrete PI Controller  Kp=Kp_iq  Ki=Ki_iq  Kaw=Kaw_iq  x0=0  Ts=Ts
  Sum : Sum  Inputs=|+-
  Sum1 : Sum  Inputs=|+-
  Sum2 : Sum  Inputs=|+--
  Sum3 : Sum  Inputs=|+++
  Sum4 : Sum  Inputs=-+|
  Sum5 : Sum  Inputs=|+-
  d-q Voltage Limiter : Subsystem  AncestorBlock=eePmsmCurrentController/PMSM Current Controller with Pre-Control/d-q Voltage Limiter  LoadFcn=ee_sli_rtmsupport( 'loadfcn', gcbh );  mask(d-q Voltage Limiter){AxisPrio=Q-axis, Ts=Ts}
      mask prompts: AxisPrio "physmod:ee:library:comments:control:eeDqVoltageLimiter:AxisPrioritization_MP"; Ts "physmod:ee:library:comments:control:eeDqVoltageLimiter:SampleTime1ForInherited_MP"
      mask help: physmod:ee:library:comments:control:eeDqVoltageLimiter:dqVoltageLimiter_MD
      settings: CopyFcn=ee_sli_rtmsupport( 'copyfcn', gcbh );  DeleteFcn=ee_sli_rtmsupport( 'deletefcn', gcbh );  ModelCloseFcn=ee_sli_rtmsupport( 'modelclosefcn', gcbh );  PostSaveFcn=ee_sli_rtmsupport( 'postsavefcn', gcbh );  PreCopyFcn=ee_sli_rtmsupport( 'precopyfcn', gcbh );  OpenFcn=ee_sli_rtmsupport( 'openfcn', gcbh );  CloseFcn=ee_sli_rtmsupport( 'closefcn', gcbh );  PreDeleteFcn=ee_sli_rtmsupport( 'predeletefcn', gcbh );
      mask Help: web(nesl_help(gcbh))
      mask TypeOptions AxisPrio: physmod:ee:library:comments:control:eeDqVoltageLimiter:D0x2DAxis_PV | physmod:ee:library:comments:control:eeDqVoltageLimiter:Q0x2DAxis_PV | physmod:ee:library:comments:control:eeDqVoltageLimiter:D0x2DQEquivalence_PV
      mask DialogControl AxisPrio Prompt: Axis prioritization
      mask DialogControl Ts Prompt: Sample time (-1 for inherited)
  vdqRef : Outport  VectorParamsAs1DForOutWhenUnconnected=off
  wires:
  VphMax/1 -> d-q Voltage Limiter/3(VphMax)
  Reset/1 -> PI id/3, PI iq/3
  idq/1 -> Demux1/1
  idqRef/1 -> Demux/1
  Sum5/1 -> PI id/2
  Demux1/2 -> Sum1/2
  Demux1/1 -> Sum/2
  d-q Voltage Limiter/2(vqRef) -> Sum4/2, Mux/2
  Sum4/1 -> PI iq/2
  Demux/2 -> Discrete Transfer Fcn3/1
  Sum3/1 -> Sum4/1, d-q Voltage Limiter/2(vqRefUnsat)
  Demux/1 -> Discrete Transfer Fcn2/1
  d-q Voltage Limiter/1(vdRef) -> Sum5/1, Mux/1
  Sum/1 -> [delta_id], PI id/1
  Sum1/1 -> [delta_iq], PI iq/1
  PI id/1 -> Sum2/1
  Discrete Transfer Fcn3/1 -> Sum1/1, [iqRef]
  PI iq/1 -> Sum3/1
  Mux/1 -> vdqRef/1
  Discrete Transfer Fcn2/1 -> [idRef], Sum/1
  Sum2/1 -> Sum5/2, d-q Voltage Limiter/1(vdRefUnsat)
  Complex Vector Decoupling/1(vdCV) -> Sum2/2
  Complex Vector Decoupling/2(vqCV) -> Sum3/2
  wElectrical/1 -> Feedforward pre-control/3(wElectrical), Complex Vector Decoupling/3(wElectrical)
  [delta_id] -> Complex Vector Decoupling/4(delta_id)
  [delta_iq] -> Complex Vector Decoupling/5(delta_iq)
  [idRef] -> Complex Vector Decoupling/1(idRef)
  [iqRef] -> Complex Vector Decoupling/2(iqRef)
  [idRef] -> Feedforward pre-control/1(idRef)
  [iqRef] -> Feedforward pre-control/2(iqRef)
  Feedforward pre-control/1(vdFF) -> Sum2/3
  Feedforward pre-control/2(vqFF) -> Sum3/3
